simulink model "auv_sonar_transmitter_payload"  (R2026a)
settings: Solver=FixedStepDiscrete  StopTime=t_mission_end  FixedStep=Ts_ping
PreLoadFcn:
  | % Self-healing path configuration for AUV Sonar Simulink Suite
  | m_file = get_param(bdroot, 'FileName');
  | if ~isempty(m_file)
  |     m_dir = fileparts(m_file);
  |     addpath(m_dir);
  |     addpath(fullfile(m_dir, '..'));
  | else
  |     if exist(fullfile(pwd, 'matlab', 'simulink'), 'dir')
  |         addpath(fullfile(pwd, 'matlab', 'simulink'));
  |         addpath(fullfile(pwd, 'matlab'));
  |     end
  | end
  | if exist('init_sonar_simulink', 'file') == 2
  |     init_sonar_simulink;
  | end
InitFcn:
  | % Self-healing path configuration for AUV Sonar Simulink Suite
  | m_file = get_param(bdroot, 'FileName');
  | if ~isempty(m_file)
  |     m_dir = fileparts(m_file);
  |     addpath(m_dir);
  |     addpath(fullfile(m_dir, '..'));
  | else
  |     if exist(fullfile(pwd, 'matlab', 'simulink'), 'dir')
  |         addpath(fullfile(pwd, 'matlab', 'simulink'));
  |         addpath(fullfile(pwd, 'matlab'));
  |     end
  | end
  | if exist('init_sonar_simulink', 'file') == 2
  |     init_sonar_simulink;
  | end
values from neighbouring files (symbols this model uses):
  Tp = 0.002    [sim_bridge_waveform.m]
undefined symbols (not defined in the file or in its folder): Ts_ping
settings Model: Creator=harsh  LastModifiedBy=harsh

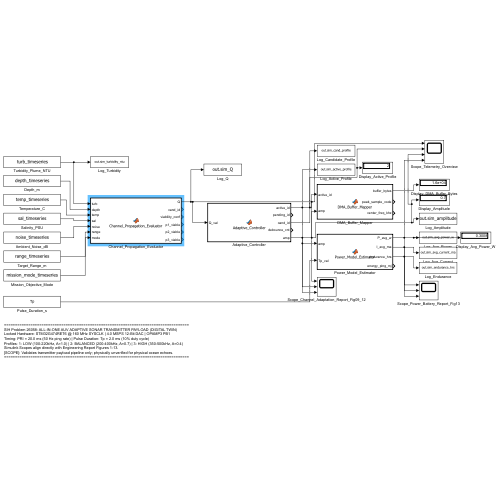
[thumbnail: Simulink's stored preview of the top-level diagram]
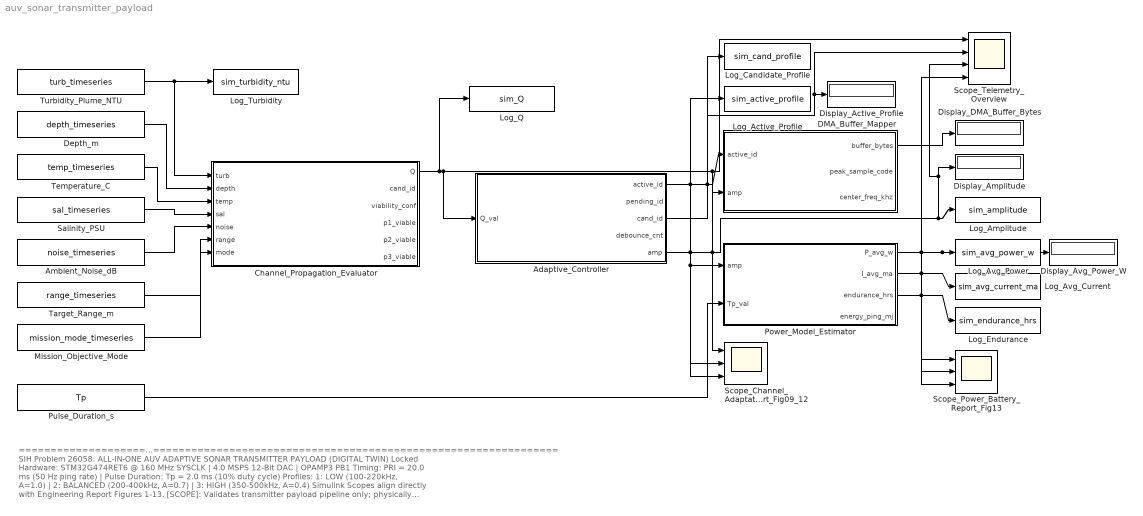
== system auv_sonar_transmitter_payload ==
  note: ====================================================================================
      | SIH Problem 26058: ALL-IN-ONE AUV ADAPTIVE SONAR TRANSMITTER PAYLOAD (DIGITAL TWIN)
      | Locked Hardware: STM32G474RET6 @ 160 MHz SYSCLK | 4.0 MSPS 12-Bit DAC | OPAMP3 PB1
      | Timing: PRI = 20.0 ms (50 Hz ping rate) | Pulse Duration: Tp = 2.0 ms (10% duty cycle)
      | Profiles: 1: LOW (100-220kHz, A=1.0) | 2: BALANCED (200-400kHz, A=0.7) | 3: HIGH (350-500kHz, A=0.4)
      | Simulink Scopes align directly with Engineering Report Figures 1-13.
      | [SCOPE]: Validates transmitter payload pipeline only; physically unverified for physical ocean echoes.
      | ====================================================================================
  Adaptive_Controller : MATLAB Function  TreatAsAtomicUnit=on
  Ambient_Noise_dB : FromWorkspace  VariableName=noise_timeseries  SampleTime=Ts_ping  OutputAfterFinalValue=Holding final value
  Channel_Propagation_Evaluator : MATLAB Function  TreatAsAtomicUnit=on
  DMA_Buffer_Mapper : MATLAB Function  TreatAsAtomicUnit=on
  Depth_m : FromWorkspace  VariableName=depth_timeseries  SampleTime=Ts_ping  OutputAfterFinalValue=Holding final value
  Display_Active_Profile : Display
  Display_Amplitude : Display
  Display_Avg_Power_W : Display
  Display_DMA_Buffer_Bytes : Display
  Log_Active_Profile : ToWorkspace  VariableName=sim_active_profile  SampleTime=-1
  Log_Amplitude : ToWorkspace  VariableName=sim_amplitude  SampleTime=-1
  Log_Avg_Current : ToWorkspace  VariableName=sim_avg_current_ma  SampleTime=-1
  Log_Avg_Power : ToWorkspace  VariableName=sim_avg_power_w  SampleTime=-1
  Log_Candidate_Profile : ToWorkspace  VariableName=sim_cand_profile  SampleTime=-1
  Log_Endurance : ToWorkspace  VariableName=sim_endurance_hrs  SampleTime=-1
  Log_Q : ToWorkspace  VariableName=sim_Q  SampleTime=-1
  Log_Turbidity : ToWorkspace  VariableName=sim_turbidity_ntu  SampleTime=-1
  Mission_Objective_Mode : FromWorkspace  VariableName=mission_mode_timeseries  SampleTime=Ts_ping  OutputAfterFinalValue=Holding final value
  Power_Model_Estimator : MATLAB Function  TreatAsAtomicUnit=on
  Pulse_Duration_s : Constant  Value=Tp
  Salinity_PSU : FromWorkspace  VariableName=sal_timeseries  SampleTime=Ts_ping  OutputAfterFinalValue=Holding final value
  Scope_Channel_Adaptation_Report_Fig09_12 : Scope  NumInputPorts=3
      settings: ActiveDisplayYMinimum=-6.1468380177264059  ActiveDisplayYMaximum=22.439350352237124
  Scope_Power_Battery_Report_Fig13 : Scope  NumInputPorts=3
      settings: ActiveDisplayYMinimum=-65.5864321876814  ActiveDisplayYMaximum=512.76972845137561
  Scope_Telemetry_Overview : Scope  NumInputPorts=4
      settings: ActiveDisplayYMinimum=-0.034956870037009646  ActiveDisplayYMaximum=2.226106318893001
  Target_Range_m : FromWorkspace  VariableName=range_timeseries  SampleTime=Ts_ping  OutputAfterFinalValue=Holding final value
  Temperature_C : FromWorkspace  VariableName=temp_timeseries  SampleTime=Ts_ping  OutputAfterFinalValue=Holding final value
  Turbidity_Plume_NTU : FromWorkspace  VariableName=turb_timeseries  SampleTime=Ts_ping  OutputAfterFinalValue=Holding final value
  wires:
  Turbidity_Plume_NTU/1 -> Channel_Propagation_Evaluator/1(turb), Log_Turbidity/1
  Depth_m/1 -> Channel_Propagation_Evaluator/2(depth)
  Temperature_C/1 -> Channel_Propagation_Evaluator/3(temp)
  Salinity_PSU/1 -> Channel_Propagation_Evaluator/4(sal)
  Ambient_Noise_dB/1 -> Channel_Propagation_Evaluator/5(noise)
  Target_Range_m/1 -> Channel_Propagation_Evaluator/6(range)
  Mission_Objective_Mode/1 -> Channel_Propagation_Evaluator/7(mode)
  Channel_Propagation_Evaluator/1(Q) -> Scope_Channel_Adaptation_Report_Fig09_12/1, Scope_Telemetry_Overview/1, Adaptive_Controller/1(Q_val), Log_Q/1
  Adaptive_Controller/1(active_id) -> Display_Active_Profile/1, Scope_Telemetry_Overview/2, DMA_Buffer_Mapper/1(active_id), Log_Active_Profile/1, Scope_Channel_Adaptation_Report_Fig09_12/2
  Adaptive_Controller/3(cand_id) -> Log_Candidate_Profile/1
  Adaptive_Controller/5(amp) -> Power_Model_Estimator/1(amp), Scope_Channel_Adaptation_Report_Fig09_12/3, Display_Amplitude/1, Scope_Telemetry_Overview/3, Log_Amplitude/1, DMA_Buffer_Mapper/2(amp)
  Pulse_Duration_s/1 -> Power_Model_Estimator/2(Tp_val)
  DMA_Buffer_Mapper/1(buffer_bytes) -> Display_DMA_Buffer_Bytes/1
  Power_Model_Estimator/1(P_avg_w) -> Log_Avg_Power/1, Display_Avg_Power_W/1, Scope_Power_Battery_Report_Fig13/1, Scope_Telemetry_Overview/4
  Power_Model_Estimator/2(I_avg_ma) -> Log_Avg_Current/1, Scope_Power_Battery_Report_Fig13/2
  Power_Model_Estimator/3(endurance_hrs) -> Log_Endurance/1, Scope_Power_Battery_Report_Fig13/3

== matlab function auv_sonar_transmitter_payload/Adaptive_Controller ==
  data: Q_val input; active_id output; pending_id output; cand_id output; debounce_cnt output; amp output
function [active_id, pending_id, cand_id, debounce_cnt, amp] = Adaptive_Controller(Q_val)
coder.extrinsic('sim_bridge_controller');
active_id = 2.0;
pending_id = 2.0;
cand_id = 2.0;
debounce_cnt = 0.0;
amp = 0.70;
[active_id, pending_id, cand_id, debounce_cnt, amp] = sim_bridge_controller(Q_val);
end

== matlab function auv_sonar_transmitter_payload/Channel_Propagation_Evaluator ==
  data: turb input; Q output; depth input; temp input; sal input; noise input; range input; mode input; cand_id output; viability_conf output; p1_viable output; p2_viable output; p3_viable output
function [Q, cand_id, viability_conf, p1_viable, p2_viable, p3_viable] = ...
    Channel_Propagation_Evaluator(turb, depth, temp, sal, noise, range, mode)
coder.extrinsic('sim_bridge_channel');
Q = 0.0;
cand_id = 1.0;
viability_conf = 0.0;
p1_viable = 0.0;
p2_viable = 0.0;
p3_viable = 0.0;
[Q, cand_id, viability_conf, p1_viable, p2_viable, p3_viable] = ...
    sim_bridge_channel(turb, depth, temp, sal, noise, range, mode);
end

== matlab function auv_sonar_transmitter_payload/Power_Model_Estimator ==
  data: amp input; P_avg_w output; Tp_val input; I_avg_ma output; endurance_hrs output; energy_ping_mj output
function [P_avg_w, I_avg_ma, endurance_hrs, energy_ping_mj] = Power_Model_Estimator(amp, Tp_val)
coder.extrinsic('sim_bridge_power');
P_avg_w = 0.0;
I_avg_ma = 0.0;
endurance_hrs = 0.0;
energy_ping_mj = 0.0;
[P_avg_w, I_avg_ma, endurance_hrs, energy_ping_mj] = sim_bridge_power(amp, Tp_val);
end

== matlab function auv_sonar_transmitter_payload/DMA_Buffer_Mapper ==
  data: active_id input; buffer_bytes output; amp input; peak_sample_code output; center_freq_khz output
function [buffer_bytes, peak_sample_code, center_freq_khz] = DMA_Buffer_Mapper(active_id, amp)
buffer_bytes = 16000.0; % 8000 samples * 2 bytes
fc = 300.0;
if active_id == 1
    fc = 160.0;
elseif active_id == 3
    fc = 425.0;
end
center_freq_khz = fc;
peak_sample_code = 2048.0 + (2047.5 * amp);
end
